simulink model "Q2_2"  (R2022b)
settings: Solver=VariableStepAuto  StartTime=0.0  StopTime=10.0  RelTol=1e-3
values from neighbouring files (symbols this model uses):
  b = 3.5077e-6    (= 3.5077e-06)    [Q2Code.m]    (also in Q3_2.m)
  J = 3.2284e-5    (= 3.2284e-05)    [Q2Code.m]    (also in Q3_1.m)
  K = 0.0274    [Q2Code.m]    (also in Q3_1.m)
  L = 2.75e-6    (= 2.75e-06)    [Q2Code.m]    (also in Q3_1.m)
  R = 4    [Q2Code.m]
settings Model: Creator=Lenovo  LastModifiedBy=Asus
settings DebuggingCC: UnconnectedInputMsg=warning  UnconnectedOutputMsg=warning  UnconnectedLineMsg=warning
settings ModelReferenceCC: EnableRefExpFcnMdlSchedulingChecks=on
settings RTWCC: DLArmComputeVersion=19.05

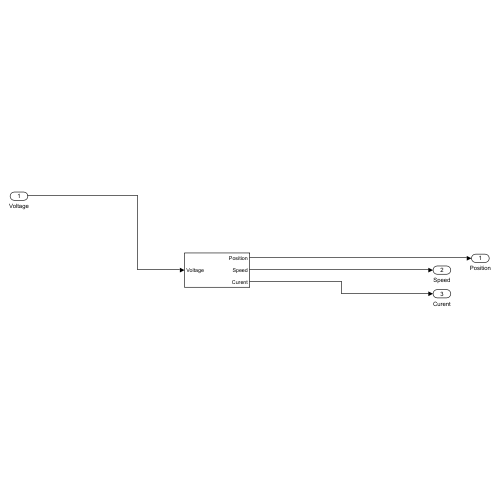
[thumbnail: Simulink's stored preview of the top-level diagram]
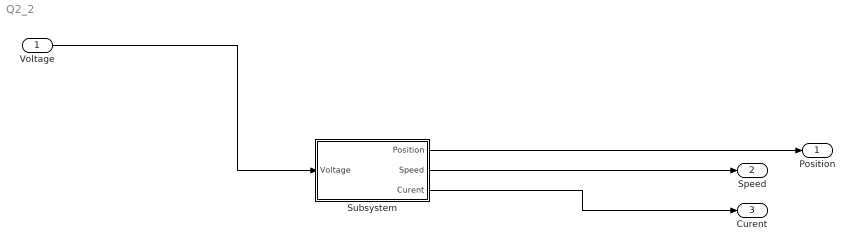
== system Q2_2 ==
  Voltage : Inport
  Subsystem : Subsystem
  Position : Outport
  Speed : Outport  Port=2
  Curent : Outport  Port=3
  wires:
  Voltage/1 -> Subsystem/1(Voltage)
  Subsystem/1(Position) -> Position/1
  Subsystem/2(Speed) -> Speed/1
  Subsystem/3(Curent) -> Curent/1

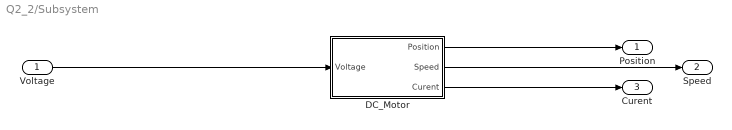
== system Q2_2/Subsystem ==
  Voltage : Inport
  DC_Motor : Subsystem
  Position : Outport
  Speed : Outport  Port=2
  Curent : Outport  Port=3
  wires:
  Voltage/1 -> DC_Motor/1(Voltage)
  DC_Motor/1(Position) -> Position/1
  DC_Motor/2(Speed) -> Speed/1
  DC_Motor/3(Curent) -> Curent/1

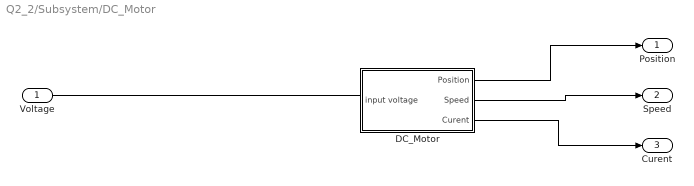
== system Q2_2/Subsystem/DC_Motor ==
  Voltage : Inport
  DC_Motor : Subsystem
  Position : Outport
  Speed : Outport  Port=2
  Curent : Outport  Port=3
  wires:
  Voltage/1 -> ?
  DC_Motor/1(Position) -> Position/1
  DC_Motor/2(Speed) -> Speed/1
  DC_Motor/3(Curent) -> Curent/1

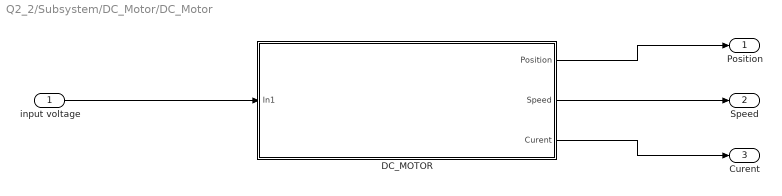
== system Q2_2/Subsystem/DC_Motor/DC_Motor ==
  input voltage : Inport
  DC_MOTOR : Subsystem
  Position : Outport
  Speed : Outport  Port=2
  Curent : Outport  Port=3
  wires:
  DC_MOTOR/1(Position) -> Position/1
  DC_MOTOR/2(Speed) -> Speed/1
  DC_MOTOR/3(Curent) -> Curent/1
  input voltage/1 -> DC_MOTOR/1(In1)

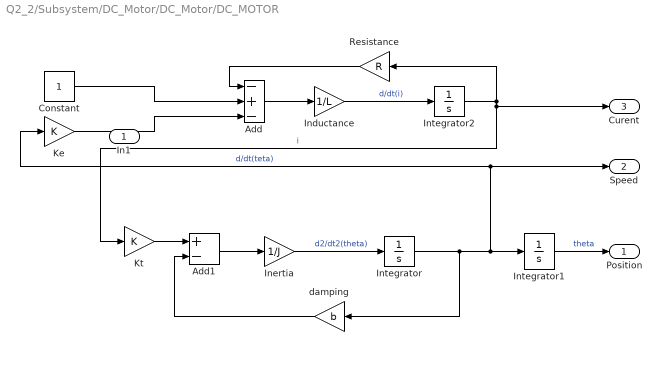
== system Q2_2/Subsystem/DC_Motor/DC_Motor/DC_MOTOR ==
  In1 : Inport
  Add : Sum  Inputs=-+-
  Add1 : Sum  Inputs=+-
  Constant : Constant
  Inductance : Gain  Gain=1/L
  Inertia : Gain  Gain=1/J  RndMeth=Convergent
  Integrator : Integrator
  Integrator1 : Integrator
  Integrator2 : Integrator
  Ke : Gain  Gain=K
  Kt : Gain  Gain=K
  Resistance : Gain  Gain=R
  damping : Gain  Gain=b
  Position : Outport
  Speed : Outport  Port=2
  Curent : Outport  Port=3
  wires:
  Inductance/1 -> Integrator2/1  "d/dt(i)"
  Add1/1 -> Inertia/1
  damping/1 -> Add1/2
  Resistance/1 -> Add/1
  Integrator2/1 -> Curent/1, Kt/1, Resistance/1  "i"
  Integrator/1 -> damping/1, Speed/1, Ke/1, Integrator1/1  "d/dt(teta)"
  Integrator1/1 -> Position/1  "theta"
  Kt/1 -> Add1/1
  Constant/1 -> Add/2
  Inertia/1 -> Integrator/1  "d2/dt2(theta)"
  Ke/1 -> Add/3
  Add/1 -> Inductance/1
